simulink model "rev_completo_with_audio_backup"  (R2018a)
settings: Solver=VariableStepAuto  StartTime=0.0  StopTime=10.0  RelTol=1e-3
libraries: dspvision x2
settings Model: Creator=Lu  LastModifiedBy=Lu

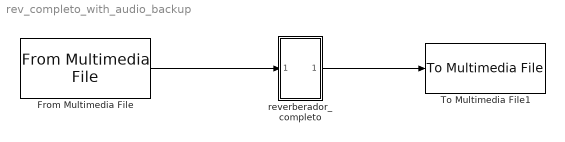
== system rev_completo_with_audio_backup ==
  From Multimedia File : dspvision/From Multimedia File  inputFilename=C:\Users\lugfe\Documents\GitHub\dsp-fpgay\TP FINAL\audio effects\dialog05.wav  loop=on  numPlays=1  outputStreams=Audio only  videoDataType=single  audioDataType=int16  inheritSampleTime=on  userDefinedSampleTime=1/30  noAudioOutput=off  isIntensityVideo=off  fourcc=RGB  colorVideoFormat=Separate color signals  outputEOF=off  dataOrg=Column-major  audioFrameSize=1  computeAudioFrameSize=off  outSamplingMode=Sample based
      settings: SourceProductBaseCode=VP
  To Multimedia File1 : dspvision/To Multimedia File  outputFilename=C:\Users\lugfe\Documents\GitHub\dsp-fpgay\TP FINAL\audio effects\rev_completo.wav  streamSelection=Audio only  videoCompressor=None (uncompressed)  audioCompressor=None (uncompressed)  imagePorts=Separate color signals  fileType=WAV  audioDatatype=Determine from input data type  fourcc=RGB  videoQuality=75  mj2000CompFactor=10
      settings: SourceProductName=Computer Vision System Toolbox  SourceProductBaseCode=VP
  "reverberador_completo " : Subsystem
  wires:
  "reverberador_completo "/1(Out1) -> To Multimedia File1/1
  From Multimedia File/1 -> "reverberador_completo "/1(In1)

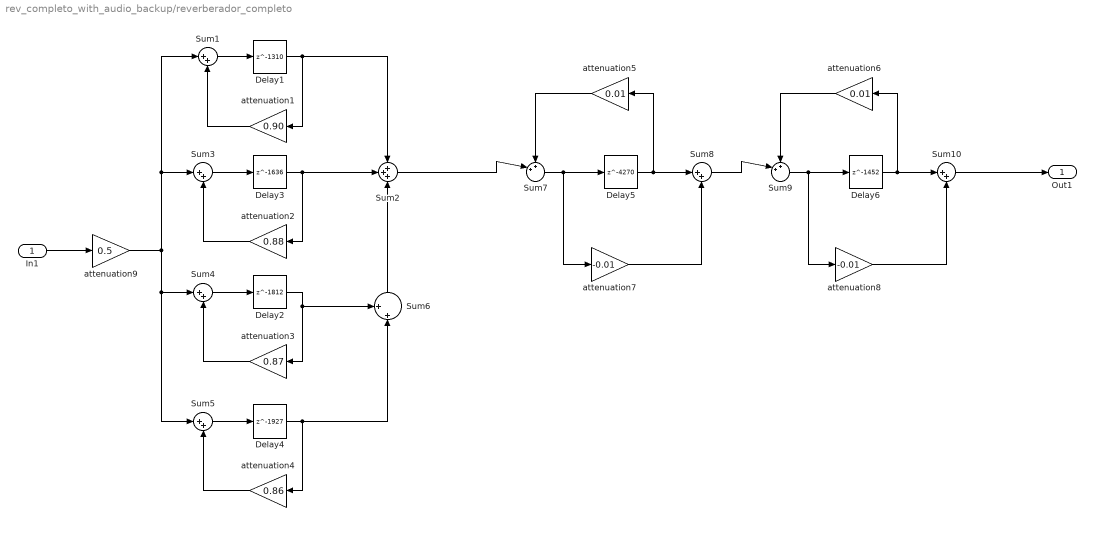
== system rev_completo_with_audio_backup/reverberador_completo  ==
  In1 : Inport  OutDataTypeStr=int16
  Delay1 : Delay  DelayLength=1310  DelayLengthUpperLimit=10000  InitialCondition=0  InputProcessing=Columns as channels (frame based)
  Delay2 : Delay  DelayLength=1812  DelayLengthUpperLimit=10000  InitialCondition=0  InputProcessing=Columns as channels (frame based)
  Delay3 : Delay  DelayLength=1636  DelayLengthUpperLimit=10000  InitialCondition=0  InputProcessing=Columns as channels (frame based)
  Delay4 : Delay  DelayLength=1927  DelayLengthUpperLimit=10000  InitialCondition=0  InputProcessing=Columns as channels (frame based)
  Delay5 : Delay  DelayLength=4270  DelayLengthUpperLimit=10000  InitialCondition=0  InputProcessing=Columns as channels (frame based)
  Delay6 : Delay  DelayLength=1452  DelayLengthUpperLimit=10000  InitialCondition=0  InputProcessing=Columns as channels (frame based)
  Sum{1,3..5,8,10} (6 alike) : Sum  Inputs=|++
  Sum2 : Sum  Inputs=+++
  Sum6 : Sum  Inputs=+|+||
  Sum7 : Sum  Inputs=++||
  Sum9 : Sum  Inputs=++||
  attenuation1 : Gain  Gain=0.90  OutDataTypeStr=int16  RndMeth=Round
  attenuation2 : Gain  Gain=0.88  OutDataTypeStr=int16  RndMeth=Round
  attenuation3 : Gain  Gain=0.87  OutDataTypeStr=int16  RndMeth=Round
  attenuation4 : Gain  Gain=0.86  OutDataTypeStr=int16  RndMeth=Round
  attenuation5 : Gain  Gain=0.01  OutDataTypeStr=int16  RndMeth=Round
  attenuation6 : Gain  Gain=0.01  OutDataTypeStr=int16  RndMeth=Round
  attenuation7 : Gain  Gain=-0.01  OutDataTypeStr=int16  RndMeth=Round
  attenuation8 : Gain  Gain=-0.01  OutDataTypeStr=int16  RndMeth=Round
  attenuation9 : Gain  Gain=0.5  OutDataTypeStr=int16  RndMeth=Round
  Out1 : Outport
  wires:
  Sum1/1 -> Delay1/1
  Sum3/1 -> Delay3/1
  attenuation2/1 -> Sum3/2
  Sum4/1 -> Delay2/1
  attenuation3/1 -> Sum4/2
  Sum5/1 -> Delay4/1
  Delay5/1 -> Sum8/1, attenuation5/1
  Sum7/1 -> Delay5/1, attenuation7/1
  attenuation5/1 -> Sum7/1
  attenuation7/1 -> Sum8/2
  attenuation6/1 -> Sum9/1
  Delay6/1 -> Sum10/1, attenuation6/1
  Sum9/1 -> Delay6/1, attenuation8/1
  attenuation8/1 -> Sum10/2
  Sum8/1 -> Sum9/2
  Sum10/1 -> Out1/1
  Sum2/1 -> Sum7/2
  Sum6/1 -> Sum2/3
  Delay1/1 -> Sum2/1, attenuation1/1
  Delay3/1 -> Sum2/2, attenuation2/1
  Delay2/1 -> Sum6/1, attenuation3/1
  Delay4/1 -> Sum6/2, attenuation4/1
  In1/1 -> attenuation9/1
  attenuation1/1 -> Sum1/2
  attenuation4/1 -> Sum5/2
  attenuation9/1 -> Sum5/1, Sum4/1, Sum1/1, Sum3/1
